simulink library "csu_rrk_rotational_kinematics_lib"  (R2014b)
settings: Solver=ode45  SolverMode=SingleTasking  StartTime=0.0  StopTime=10.0  RelTol=1e-3
libraries: util_quat_lib x3, util_info_lib x1, util_common_lib x1
settings Model: ExtModeAutoUpdateStatusClock=off  Creator=daniloviazzo  LastModifiedBy=mstewart

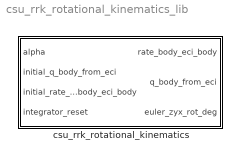
== system csu_rrk_rotational_kinematics_lib ==
  csu_rrk_rotational_kinematics : Subsystem

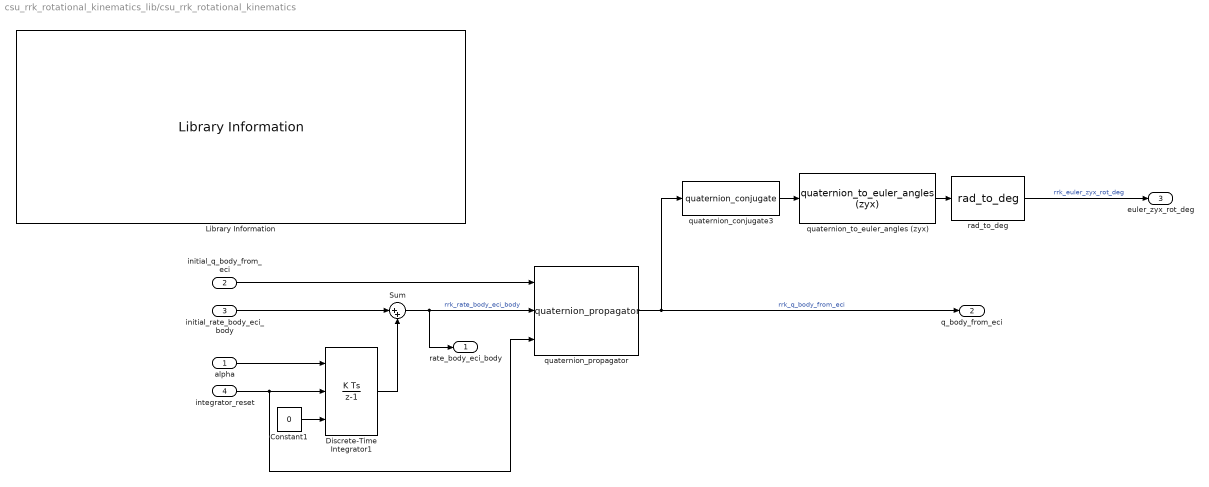
== system csu_rrk_rotational_kinematics_lib/csu_rrk_rotational_kinematics ==
  alpha : Inport
  initial_q_body_from_eci : Inport  Port=2
  initial_rate_body_eci_body : Inport  Port=3
  integrator_reset : Inport  Port=4
  Constant1 : Constant  Value=0
  Discrete-Time Integrator1 : DiscreteIntegrator  ExternalReset=rising  InitialConditionSource=external  InitialConditionSetting=Compatibility  SampleTime=-1
  Library Information : util_info_lib/Library Information  owner='NONE'
  Sum : Sum  Inputs=|++
  quaternion_conjugate3 : util_quat_lib/quaternion_conjugate  SystemSampleTime=-1
  quaternion_propagator : util_quat_lib/quaternion_propagator  SystemSampleTime=-1
  quaternion_to_euler_angles (zyx) : util_quat_lib/quaternion_to_euler_angles (zyx)  SystemSampleTime=-1
  rad_to_deg : util_common_lib/rad_to_deg  SystemSampleTime=-1
  rate_body_eci_body : Outport
  q_body_from_eci : Outport  Port=2
  euler_zyx_rot_deg : Outport  Port=3
  wires:
  quaternion_conjugate3/1 -> quaternion_to_euler_angles (zyx)/1
  rad_to_deg/1 -> euler_zyx_rot_deg/1  "rrk_euler_zyx_rot_deg"
  quaternion_to_euler_angles (zyx)/1 -> rad_to_deg/1
  initial_q_body_from_eci/1 -> quaternion_propagator/1
  Sum/1 -> rate_body_eci_body/1, quaternion_propagator/2  "rrk_rate_body_eci_body"
  Discrete-Time Integrator1/1 -> Sum/2
  initial_rate_body_eci_body/1 -> Sum/1
  alpha/1 -> Discrete-Time Integrator1/1
  Constant1/1 -> Discrete-Time Integrator1/3
  integrator_reset/1 -> Discrete-Time Integrator1/2, quaternion_propagator/3
  quaternion_propagator/1 -> q_body_from_eci/1, quaternion_conjugate3/1  "rrk_q_body_from_eci"
